simulink model "walker_fixedFoot"  (R2021a)
settings: Solver=VariableStepAuto  StartTime=0.0  StopTime=total_time  RelTol=1e-3
values from neighbouring files (symbols this model uses):
  I_thigh_xx = thigh.mass/20 * (thigh.depth^2 + thigh.height^2)    [createWalkerWithFixedStanceFootModel.m]
  I_thigh_yy = thigh.mass/20 * (thigh.width^2 + thigh.height^2)    [createWalkerWithFixedStanceFootModel.m]
  I_thigh_zz = thigh.mass/20 * (thigh.depth^2 + thigh.width^2)    [createWalkerWithFixedStanceFootModel.m]
  I_trunk_xx = trunk.mass/20 * (trunk.depth^2 + trunk.height^2)    [createWalkerWithFixedStanceFootModel.m]
  I_trunk_yy = trunk.mass/20 * (trunk.width^2 + trunk.height^2)    [createWalkerWithFixedStanceFootModel.m]
  I_trunk_zz = trunk.mass/20 * (trunk.depth^2 + trunk.width^2)    [createWalkerWithFixedStanceFootModel.m]
  shank_com_from_ankle = geometry.ankle_to_knee_z / 2    [setBiomechanicsParameters.m]
  shank_com_from_knee = geometry.ankle_to_knee_z / 2    [setBiomechanicsParameters.m]
  tau = inverseDynamics(model, theta_init, theta_dot_init)    [initialize.m]
  theta_dot_init = [0; 0; 0; 0; 0; 0]    [initialize.m]
  theta_init = [IC.left_ankle_angle; IC.left_knee_angle; IC.left_hip_angle; IC.right_hip_angle; IC.right_knee_angle; IC.right_ankle_angle]    [initialize.m]
  thigh_com_from_hip = geometry.knee_to_hip_z / 2    [setBiomechanicsParameters.m]
  thigh_com_from_knee = geometry.knee_to_hip_z / 2    [setBiomechanicsParameters.m]
undefined symbols (not defined in the file or in its folder): foot, geometry, head, shank, thigh, trunk, X, Y, Z
libraries: sm_lib x56, nesl_utility x25
(part 1 of 2)
settings Model: Creator=reimajbi  LastModifiedBy=reimajbi

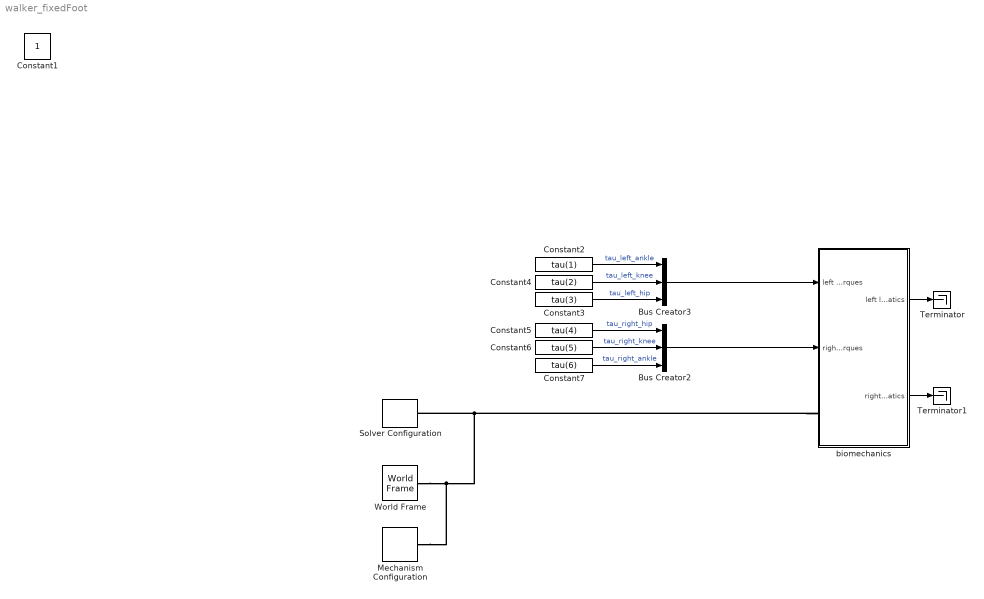
== system walker_fixedFoot ==
  Bus Creator2 : BusCreator  Inputs=3
  Bus Creator3 : BusCreator  Inputs=3
  Constant2 : Constant  Value=tau(1)
  Constant3 : Constant  Value=tau(3)
  Constant4 : Constant  Value=tau(2)
  Constant5 : Constant  Value=tau(4)
  Constant6 : Constant  Value=tau(5)
  Constant7 : Constant  Value=tau(6)
  Mechanism Configuration : sm_lib/Utilities/Mechanism Configuration  UniformGravity=Constant  GravityVector=[0 0 -9.80665]  GravityVectorUnits=m/s^2  GravityUnits=m/s^2  LinearizationDelta=0.001  JointModeTransitionNonlinearIterations=2
  Solver Configuration : nesl_utility/Solver Configuration  PhysicalDomain=network_engine_domain  SubClassName=solver  LeftPortType=input  RightPortType=generic  Tones=[]  Harmonics=[]  SimulateNoise=off  Profile=off  UseLocalSampling=off  EnableSwitchedLinearOptims=on  FrequencyDomain=off  UseCCode=off  RelTol=0.001  AbsTol=1e-06  MinStep=1e-09  ToWorkspace=off  RevertToSquareIcSolve=off  NumHomotopyIterations=100  PhasorMode=off  PhasorModeNumHarmonics=1  DoDC=off  ResidualTolerance=1e-09  UseLocalSolver=off  LocalSolverChoice=NE_BACKWARD_EULER_ADVANCER  LocalSolverSampleTime=0.001  DoFixedCost=off  MaxNonlinIter=3  MaxModeIter=2  ComputeImpulses=off  ImpulseIterations=2  LinearAlgebra=Sparse  EquationFormulation=NE_TIME_EF  DelaysMemoryBudget=1024  AutomaticFiltering=on  FilteringTimeConstant=0.001  PartitionStorageMethod=AS_NEEDED  PartitionMemoryBudget=1024  PartitionMethod=FAST
      settings: SourceProductBaseCode=PW,SS
  Terminator : Terminator
  Terminator1 : Terminator
  World Frame : sm_lib/Frames and Transforms/World Frame
  biomechanics : Subsystem
  Constant1 : Constant  IOType=siggen
  wires:
  Constant3/1 -> Bus Creator3/3  "tau_left_hip"
  Constant4/1 -> Bus Creator3/2  "tau_left_knee"
  Constant2/1 -> Bus Creator3/1  "tau_left_ankle"
  Constant5/1 -> Bus Creator2/1  "tau_right_hip"
  Constant6/1 -> Bus Creator2/2  "tau_right_knee"
  Constant7/1 -> Bus Creator2/3  "tau_right_ankle"
  Bus Creator3/1 -> biomechanics/1(left leg torques)
  Bus Creator2/1 -> biomechanics/2(right leg torques)
  biomechanics/1(left leg kinematics) -> Terminator/1
  biomechanics/2(right leg kinematics) -> Terminator1/1
  connections:
  World Frame/RConn1 -- biomechanics/LConn1 -- Solver Configuration/RConn1 -- Mechanism Configuration/RConn1
